simulink model "raibert_controller_walking"  (R2018b)
settings: Solver=FixedStepDiscrete  StartTime=0.0  StopTime=inf  FixedStep=sample_time  RelTol=1e-3
InitFcn:
  | warning off all
undefined symbols (not defined in the file or in its folder): ctrl, DiscIntNeverNeededParam, Discrete, initial_dx_estimate, initial_dy_estimate, initial_dz_estimate, initial_z_estimate, sample_time, Time
libraries: simulink x28, ctrlSharedLib x7
(part 3 of 4)

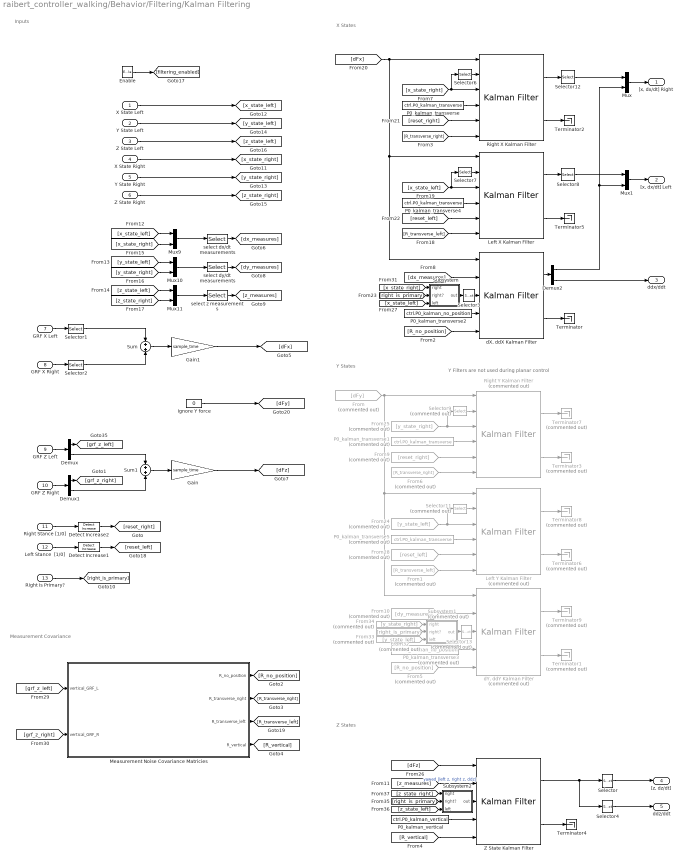
== system raibert_controller_walking/Behavior/Filtering/Kalman Filtering ==
  note: Y Filters are not used during planar control
  note: Inputs
  note: X States
  note: Y States
  note: Z States
  note: Measurement Covariance
  X State Left : Inport  SampleTime=sample_time
  Y State Left : Inport  Port=2  SampleTime=sample_time
  Z State Left : Inport  Port=3  SampleTime=sample_time
  X State Right : Inport  Port=4  SampleTime=sample_time
  Y State Right : Inport  Port=5  SampleTime=sample_time
  Z State Right : Inport  Port=6  SampleTime=sample_time
  GRF X Left : Inport  Port=7  SampleTime=sample_time
  GRF X Right : Inport  Port=8  SampleTime=sample_time
  GRF Z Left : Inport  Port=9  SampleTime=sample_time
  GRF Z Right : Inport  Port=10  SampleTime=sample_time
  Right Stance [1/0] : Inport  Port=11  PortDimensions=1  SampleTime=sample_time
  Left Stance  [1/0] : Inport  Port=12  PortDimensions=1  SampleTime=sample_time
  Right Is Primary? : Inport  Port=13  SampleTime=sample_time
  Enable : EnablePort  StatesWhenEnabling=reset  ShowOutputPort=on
  Demux : Demux  Outputs=2
  Demux1 : Demux  Outputs=2
  Demux2 : Demux  Outputs=2
  Detect Increase1 : simulink/Logic and Bit Operations/Detect Increase  vinit=0.0  OutDataTypeStr=boolean
  Detect Increase2 : simulink/Logic and Bit Operations/Detect Increase  vinit=0.0  OutDataTypeStr=boolean
  From : From  Commented=on  GotoTag=dFy
  From1 : From  Commented=on  GotoTag=R_transverse_left
  From10 : From  Commented=on  GotoTag=dy_measures
  From24 : From  Commented=on  GotoTag=y_state_left
  From25 : From  Commented=on  GotoTag=y_state_right
  From28 : From  Commented=on  GotoTag=reset_left
  From32 : From  Commented=on  GotoTag=right_is_primary
  From33 : From  Commented=on  GotoTag=y_state_left
  From34 : From  Commented=on  GotoTag=y_state_right
  From5 : From  Commented=on  GotoTag=R_no_position
  From6 : From  Commented=on  GotoTag=R_transverse_right
  From9 : From  Commented=on  GotoTag=reset_right
  Gain : Gain  Gain=sample_time
  Gain1 : Gain  Gain=sample_time
  Ignore Y force : Constant  Value=0
  Left X Kalman Filter : ctrlSharedLib/Kalman Filter  TimeDomain=Discrete-Time  UseCurrentEstimator=on  ModelSource=Individual A, B, C, D matrices  ModelSourceVariable=A_kf  A=ctrl.A_kalman_3rd_order  B=ctrl.B_kalman_3rd_order  C=ctrl.C_kalman_transverse  D=0  NumberOfStates=2  NumberOfInputs=1  NumberOfOutputs=2  InitialEstimateSource=Input port  X0=initial_dx_estimate  P0=P0_kalman_transverse  UseK=off  UseGH=on  NumberOfProcessNoiseInputs=1  G=ctrl.G_kalman_transverse  TimeInvariantG=on  H=0  TimeInvariantH=on  Q=ctrl.Q_kalman_GRFx_difference*sample_time  TimeInvariantQ=on  R=1  TimeInvariantR=off  N=0  TimeInvariantN=on  AddInputPort=on  AddEnablePort=off  ExternalReset=Rising  OutputEstimatedY=off  OutputP=on  Ts=sample_time
      settings: SourceProductBaseCode=CT
  Left Y Kalman Filter : ctrlSharedLib/Kalman Filter  Commented=on  TimeDomain=Discrete-Time  UseCurrentEstimator=on  ModelSource=Individual A, B, C, D matrices  ModelSourceVariable=A_kf  A=ctrl.A_kalman_3rd_order  B=ctrl.B_kalman_3rd_order  C=ctrl.C_kalman_transverse  D=0  NumberOfStates=2  NumberOfInputs=1  NumberOfOutputs=2  InitialEstimateSource=Input port  X0=initial_dy_estimate  P0=P0_kalman_transverse  UseK=off  UseGH=on  NumberOfProcessNoiseInputs=1  G=ctrl.G_kalman_transverse  TimeInvariantG=on  H=0  TimeInvariantH=on  Q=ctrl.Q_kalman_GRFy_difference*sample_time  TimeInvariantQ=on  R=1  TimeInvariantR=off  N=0  TimeInvariantN=on  AddInputPort=on  AddEnablePort=off  ExternalReset=Rising  OutputEstimatedY=off  OutputP=on  Ts=sample_time
      settings: SourceProductBaseCode=CT
  Measurement Noise Covariance Matricies : MATLAB Function  TreatAsAtomicUnit=on
  Mux{,1,9..11} (5 alike) : Mux  Inputs=2
  P0_kalman_transverse : Constant  Value=ctrl.P0_kalman_transverse
  P0_kalman_transverse1 : Constant  Commented=on  Value=ctrl.P0_kalman_transverse
  P0_kalman_transverse2 : Constant  Value=ctrl.P0_kalman_no_position
  P0_kalman_transverse3 : Constant  Commented=on  Value=ctrl.P0_kalman_no_position
  P0_kalman_transverse4 : Constant  Value=ctrl.P0_kalman_transverse
  P0_kalman_transverse5 : Constant  Commented=on  Value=ctrl.P0_kalman_transverse
  P0_kalman_vertical : Constant  Value=ctrl.P0_kalman_vertical
  Right X Kalman Filter : ctrlSharedLib/Kalman Filter  TimeDomain=Discrete-Time  UseCurrentEstimator=on  ModelSource=Individual A, B, C, D matrices  ModelSourceVariable=A_kf  A=ctrl.A_kalman_3rd_order  B=ctrl.B_kalman_3rd_order  C=ctrl.C_kalman_transverse  D=0  NumberOfStates=2  NumberOfInputs=1  NumberOfOutputs=2  InitialEstimateSource=Input port  X0=initial_dx_estimate  P0=P0_kalman_transverse  UseK=off  UseGH=on  NumberOfProcessNoiseInputs=1  G=ctrl.G_kalman_transverse  TimeInvariantG=on  H=0  TimeInvariantH=on  Q=ctrl.Q_kalman_GRFx_difference*sample_time  TimeInvariantQ=on  R=1  TimeInvariantR=off  N=0  TimeInvariantN=on  AddInputPort=on  AddEnablePort=off  ExternalReset=Rising  OutputEstimatedY=off  OutputP=on  Ts=sample_time
      settings: SourceProductBaseCode=CT
  Right Y Kalman Filter : ctrlSharedLib/Kalman Filter  Commented=on  TimeDomain=Discrete-Time  UseCurrentEstimator=on  ModelSource=Individual A, B, C, D matrices  ModelSourceVariable=A_kf  A=ctrl.A_kalman_3rd_order  B=ctrl.B_kalman_3rd_order  C=ctrl.C_kalman_transverse  D=0  NumberOfStates=2  NumberOfInputs=1  NumberOfOutputs=2  InitialEstimateSource=Input port  X0=initial_dy_estimate  P0=P0_kalman_transverse  UseK=off  UseGH=on  NumberOfProcessNoiseInputs=1  G=ctrl.G_kalman_transverse  TimeInvariantG=on  H=0  TimeInvariantH=on  Q=ctrl.Q_kalman_GRFy_difference*sample_time  TimeInvariantQ=on  R=1  TimeInvariantR=off  N=0  TimeInvariantN=on  AddInputPort=on  AddEnablePort=off  ExternalReset=Rising  OutputEstimatedY=off  OutputP=on  Ts=sample_time
      settings: SourceProductBaseCode=CT
  Selector : Selector  InputPortWidth=3  IndexOptions=Index vector (dialog)  Indices=[1 2]  OutputSizes=1
  Selector1 : Selector  InputPortWidth=2  IndexOptions=Index vector (dialog)  Indices=[2]  OutputSizes=1
  Selector11 : Selector  Commented=on  InputPortWidth=3  IndexOptions=Index vector (dialog)  Indices=[1 3]  OutputSizes=1
  Selector12 : Selector  InputPortWidth=3  IndexOptions=Index vector (dialog)  Indices=[1]  OutputSizes=1
  Selector13 : Selector  Commented=on  InputPortWidth=3  IndexOptions=Index vector (dialog)  Indices=[2 3]  OutputSizes=1
  Selector2 : Selector  InputPortWidth=2  IndexOptions=Index vector (dialog)  Indices=[2]  OutputSizes=1
  Selector3 : Selector  InputPortWidth=3  IndexOptions=Index vector (dialog)  Indices=[2 3]  OutputSizes=1
  Selector4 : Selector  InputPortWidth=3  IndexOptions=Index vector (dialog)  Indices=[3]  OutputSizes=1
  Selector6 : Selector  InputPortWidth=3  IndexOptions=Index vector (dialog)  Indices=[1 3]  OutputSizes=1
  Selector7 : Selector  InputPortWidth=3  IndexOptions=Index vector (dialog)  Indices=[1 3]  OutputSizes=1
  Selector8 : Selector  InputPortWidth=3  IndexOptions=Index vector (dialog)  Indices=[1]  OutputSizes=1
  Selector9 : Selector  Commented=on  InputPortWidth=3  IndexOptions=Index vector (dialog)  Indices=[1 3]  OutputSizes=1
  Subsystem : Subsystem
  Subsystem1 : Subsystem  Commented=on
  Subsystem2 : Subsystem
  Sum : Sum  Inputs=+|+
  Sum1 : Sum  Inputs=+|+
  Terminator{,2,4..5} (4 alike) : Terminator
  Terminator{1,3,6..9} (6 alike) : Terminator  Commented=on
  Z State Kalman Filter : ctrlSharedLib/Kalman Filter  TimeDomain=Discrete-Time  UseCurrentEstimator=on  ModelSource=Individual A, B, C, D matrices  ModelSourceVariable=A_kf  A=ctrl.A_kalman_3rd_order  B=ctrl.B_kalman_3rd_order  C=ctrl.C_kalman_vertical  D=0  NumberOfStates=2  NumberOfInputs=1  NumberOfOutputs=2  InitialEstimateSource=Input port  X0=[initial_z_estimate; initial_dz_estimate]  P0=P0_kalman_vertical  UseK=off  UseGH=on  NumberOfProcessNoiseInputs=1  G=ctrl.G_kalman_vertical  TimeInvariantG=on  H=0  TimeInvariantH=on  Q=ctrl.Q_kalman_GRFz_difference*sample_time  TimeInvariantQ=on  R=1  TimeInvariantR=off  N=0  TimeInvariantN=on  AddInputPort=on  AddEnablePort=off  OutputEstimatedY=off  OutputP=on  Ts=sample_time
      settings: SourceProductBaseCode=CT
  "dX, ddX Kalman Filter" : ctrlSharedLib/Kalman Filter  TimeDomain=Discrete-Time  UseCurrentEstimator=on  ModelSource=Individual A, B, C, D matrices  ModelSourceVariable=A_kf  A=ctrl.A_kalman_2nd_order  B=ctrl.B_kalman_2nd_order  C=ctrl.C_kalman_no_position  D=0  NumberOfStates=2  NumberOfInputs=1  NumberOfOutputs=2  InitialEstimateSource=Input port  X0=initial_dx_estimate  P0=P0_kalman_transverse  UseK=off  UseGH=on  NumberOfProcessNoiseInputs=1  G=ctrl.G_kalman_no_position  TimeInvariantG=on  H=0  TimeInvariantH=on  Q=ctrl.Q_kalman_GRFx_difference*sample_time  TimeInvariantQ=on  R=1  TimeInvariantR=off  N=0  TimeInvariantN=on  AddInputPort=on  AddEnablePort=off  OutputEstimatedY=off  OutputP=on  Ts=sample_time
      settings: SourceProductBaseCode=CT
  "dY, ddY Kalman Filter" : ctrlSharedLib/Kalman Filter  Commented=on  TimeDomain=Discrete-Time  UseCurrentEstimator=on  ModelSource=Individual A, B, C, D matrices  ModelSourceVariable=A_kf  A=ctrl.A_kalman_2nd_order  B=ctrl.B_kalman_2nd_order  C=ctrl.C_kalman_no_position  D=0  NumberOfStates=2  NumberOfInputs=1  NumberOfOutputs=2  InitialEstimateSource=Input port  X0=initial_dx_estimate  P0=P0_kalman_transverse  UseK=off  UseGH=on  NumberOfProcessNoiseInputs=1  G=ctrl.G_kalman_no_position  TimeInvariantG=on  H=0  TimeInvariantH=on  Q=ctrl.Q_kalman_GRFx_difference*sample_time  TimeInvariantQ=on  R=1  TimeInvariantR=off  N=0  TimeInvariantN=on  AddInputPort=on  AddEnablePort=off  OutputEstimatedY=off  OutputP=on  Ts=sample_time
      settings: SourceProductBaseCode=CT
  select dx/dt measurements : Selector  InputPortWidth=6  IndexOptions=Index vector (dialog)  Indices=[2 5 6]  OutputSizes=1
  select dy/dt measurements : Selector  InputPortWidth=6  IndexOptions=Index vector (dialog)  Indices=[2 5 6]  OutputSizes=1
  select z measurements : Selector  InputPortWidth=6  IndexOptions=Index vector (dialog)  Indices=[1 4 6]  OutputSizes=1
  "[x, dx/dt] Right" : Outport
  "[x, dx/dt] Left" : Outport  Port=2
  ddx/ddt : Outport  Port=3
  "[z, dz/dt]" : Outport  Port=4
  ddz/ddt : Outport  Port=5
  wires:
  [R_no_position] -> "dX, ddX Kalman Filter"/5
  P0_kalman_transverse2/1 -> "dX, ddX Kalman Filter"/4
  Subsystem/1(out) -> Selector3/1
  [dx_measures] -> "dX, ddX Kalman Filter"/2
  Z State Kalman Filter/1 -> Selector4/1, Selector/1
  [z_measures] -> Z State Kalman Filter/2  "yawed [left z, right z, ddz]"
  [R_vertical] -> Z State Kalman Filter/5
  [grf_z_right] -> Measurement Noise Covariance Matricies/2(vertical_GRF_R)
  [grf_z_left] -> Measurement Noise Covariance Matricies/1(vertical_GRF_L)
  P0_kalman_transverse1/1 -> Right Y Kalman Filter/4
  [dFz] -> Z State Kalman Filter/1
  P0_kalman_transverse/1 -> Right X Kalman Filter/4
  [dFx] -> Right X Kalman Filter/1, Left X Kalman Filter/1, "dX, ddX Kalman Filter"/1
  Right X Kalman Filter/1 -> Selector12/1
  "dX, ddX Kalman Filter"/2 -> Terminator/1
  [R_transverse_right] -> Right X Kalman Filter/6
  P0_kalman_vertical/1 -> Z State Kalman Filter/4
  "dY, ddY Kalman Filter"/2 -> Terminator1/1
  Subsystem1/1(out) -> Selector13/1
  P0_kalman_transverse3/1 -> "dY, ddY Kalman Filter"/4
  From10/1 -> "dY, ddY Kalman Filter"/2
  Measurement Noise Covariance Matricies/1(R_no_position) -> [R_no_position]
  Measurement Noise Covariance Matricies/2(R_transverse_right) -> [R_transverse_right]
  Measurement Noise Covariance Matricies/4(R_vertical) -> [R_vertical]
  From5/1 -> "dY, ddY Kalman Filter"/5
  From6/1 -> Right Y Kalman Filter/6
  Right Is Primary?/1 -> [right_is_primary]
  Y State Right/1 -> [y_state_right]
  [x_state_left] -> Mux9/1
  [x_state_right] -> Mux9/2
  [y_state_left] -> Mux10/1
  [y_state_right] -> Mux10/2
  [z_state_left] -> Mux11/1
  [z_state_right] -> Mux11/2
  Mux9/1 -> select dx/dt measurements/1
  Mux10/1 -> select dy/dt measurements/1
  Mux11/1 -> select z measurements/1
  select dx/dt measurements/1 -> [dx_measures]
  select dy/dt measurements/1 -> [dy_measures]
  select z measurements/1 -> [z_measures]
  Right X Kalman Filter/2 -> Terminator2/1
  Right Y Kalman Filter/2 -> Terminator3/1
  Z State Kalman Filter/2 -> Terminator4/1
  Enable/1 -> [filtering_enabled]
  [x_state_right] -> Selector6/1, Right X Kalman Filter/3
  Selector6/1 -> Right X Kalman Filter/2
  Selector7/1 -> Left X Kalman Filter/2
  [x_state_left] -> Left X Kalman Filter/3, Selector7/1
  [R_transverse_left] -> Left X Kalman Filter/6
  P0_kalman_transverse4/1 -> Left X Kalman Filter/4
  Left X Kalman Filter/1 -> Selector8/1
  Left X Kalman Filter/2 -> Terminator5/1
  [reset_right] -> Right X Kalman Filter/5
  [reset_left] -> Left X Kalman Filter/5
  From9/1 -> Right Y Kalman Filter/5
  From25/1 -> Selector9/1, Right Y Kalman Filter/3
  Selector9/1 -> Right Y Kalman Filter/2
  Selector11/1 -> Left Y Kalman Filter/2
  From24/1 -> Left Y Kalman Filter/3, Selector11/1
  From28/1 -> Left Y Kalman Filter/5
  Left Y Kalman Filter/2 -> Terminator6/1
  From1/1 -> Left Y Kalman Filter/6
  From/1 -> Right Y Kalman Filter/1, Left Y Kalman Filter/1, "dY, ddY Kalman Filter"/1
  P0_kalman_transverse5/1 -> Left Y Kalman Filter/4
  Right Stance [1/0]/1 -> Detect Increase2/1
  Left Stance  [1/0]/1 -> Detect Increase1/1
  Detect Increase1/1 -> [reset_left]
  Detect Increase2/1 -> [reset_right]
  GRF X Left/1 -> Selector1/1
  GRF X Right/1 -> Selector2/1
  Sum/1 -> Gain1/1
  Measurement Noise Covariance Matricies/3(R_transverse_left) -> [R_transverse_left]
  GRF Z Left/1 -> Demux/1
  GRF Z Right/1 -> Demux1/1
  Sum1/1 -> Gain/1
  Demux/1 -> [grf_z_left]
  Demux1/1 -> [grf_z_right]
  Selector1/1 -> Sum/1
  Selector2/1 -> Sum/2
  Demux/2 -> Sum1/1
  Demux1/2 -> Sum1/2
  Gain/1 -> [dFz]
  Gain1/1 -> [dFx]
  Ignore Y force/1 -> [dFy]
  Mux/1 -> "[x, dx/dt] Right"/1
  Selector12/1 -> Mux/1
  Mux1/1 -> "[x, dx/dt] Left"/1
  Selector8/1 -> Mux1/1
  Right Y Kalman Filter/1 -> Terminator7/1
  Left Y Kalman Filter/1 -> Terminator8/1
  "dY, ddY Kalman Filter"/1 -> Terminator9/1
  [x_state_right] -> Subsystem/1(right)
  [right_is_primary] -> Subsystem/2(right?)
  [x_state_left] -> Subsystem/3(left)
  From32/1 -> Subsystem1/2(right?)
  From34/1 -> Subsystem1/1(right)
  From33/1 -> Subsystem1/3(left)
  Selector13/1 -> "dY, ddY Kalman Filter"/3
  Selector3/1 -> "dX, ddX Kalman Filter"/3
  [right_is_primary] -> Subsystem2/2(right?)
  [z_state_right] -> Subsystem2/1(right)
  [z_state_left] -> Subsystem2/3(left)
  Subsystem2/1(out) -> Z State Kalman Filter/3
  Selector/1 -> "[z, dz/dt]"/1
  Demux2/1 -> Mux1/2, Mux/2
  Demux2/2 -> ddx/ddt/1
  Selector4/1 -> ddz/ddt/1
  "dX, ddX Kalman Filter"/1 -> Demux2/1
  Z State Left/1 -> [z_state_left]
  Y State Left/1 -> [y_state_left]
  X State Left/1 -> [x_state_left]
  Z State Right/1 -> [z_state_right]
  X State Right/1 -> [x_state_right]

== system raibert_controller_walking/Behavior/Filtering/Subsystem2 ==
  right : Inport
  right? : Inport  Port=2
  left : Inport  Port=3
  Switch : Switch  Criteria=u2 ~= 0
  out : Outport
  wires:
  right/1 -> Switch/1
  right?/1 -> Switch/2
  left/1 -> Switch/3
  Switch/1 -> out/1

== system raibert_controller_walking/Behavior/Raibert Controller/Hold Value ==
  In : Inport
  Enable : EnablePort
  Out : Outport  InitialOutput=0
  wires:
  In/1 -> Out/1

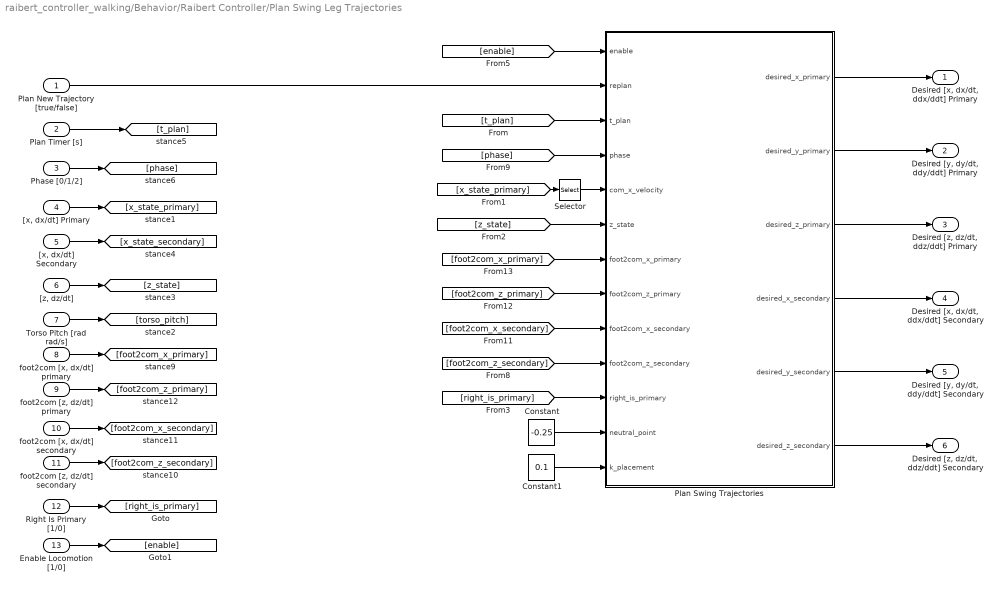
== system raibert_controller_walking/Behavior/Raibert Controller/Plan Swing Leg Trajectories ==
  Plan New Trajectory [true/false] : Inport
  Plan Timer [s] : Inport  Port=2
  Phase [0/1/2] : Inport  Port=3
  "[x, dx/dt] Primary" : Inport  Port=4
  "[x, dx/dt] Secondary" : Inport  Port=5
  "[z, dz/dt]" : Inport  Port=6
  Torso Pitch [rad rad/s] : Inport  Port=7
  "foot2com [x, dx/dt] primary" : Inport  Port=8
  "foot2com [z, dz/dt] primary" : Inport  Port=9
  "foot2com [x, dx/dt] secondary" : Inport  Port=10
  "foot2com [z, dz/dt] secondary" : Inport  Port=11
  Right Is Primary [1/0] : Inport  Port=12
  Enable Locomotion [1/0] : Inport  Port=13
  Constant : Constant  Value=-0.25
  Constant1 : Constant  Value=0.1
  Plan Swing Trajectories : MATLAB Function  TreatAsAtomicUnit=on
  Selector : Selector  InputPortWidth=2  IndexOptions=Index vector (dialog)  Indices=[2]  OutputSizes=1
  "Desired [x, dx/dt, ddx/ddt] Primary" : Outport
  "Desired [y, dy/dt, ddy/ddt] Primary" : Outport  Port=2
  "Desired [z, dz/dt, ddz/ddt] Primary" : Outport  Port=3
  "Desired [x, dx/dt, ddx/ddt] Secondary" : Outport  Port=4
  "Desired [y, dy/dt, ddy/ddt] Secondary" : Outport  Port=5
  "Desired [z, dz/dt, ddz/ddt] Secondary" : Outport  Port=6
  wires:
  Plan Timer [s]/1 -> [t_plan]
  Phase [0/1/2]/1 -> [phase]
  "[x, dx/dt] Secondary"/1 -> [x_state_secondary]
  Plan New Trajectory [true/false]/1 -> Plan Swing Trajectories/2(replan)
  Torso Pitch [rad rad/s]/1 -> [torso_pitch]
  "[x, dx/dt] Primary"/1 -> [x_state_primary]
  "[z, dz/dt]"/1 -> [z_state]
  Plan Swing Trajectories/1(desired_x_primary) -> "Desired [x, dx/dt, ddx/ddt] Primary"/1
  Plan Swing Trajectories/2(desired_y_primary) -> "Desired [y, dy/dt, ddy/ddt] Primary"/1
  Plan Swing Trajectories/3(desired_z_primary) -> "Desired [z, dz/dt, ddz/ddt] Primary"/1
  Plan Swing Trajectories/4(desired_x_secondary) -> "Desired [x, dx/dt, ddx/ddt] Secondary"/1
  Plan Swing Trajectories/5(desired_y_secondary) -> "Desired [y, dy/dt, ddy/ddt] Secondary"/1
  Plan Swing Trajectories/6(desired_z_secondary) -> "Desired [z, dz/dt, ddz/ddt] Secondary"/1
  Right Is Primary [1/0]/1 -> [right_is_primary]
  Enable Locomotion [1/0]/1 -> [enable]
  "foot2com [x, dx/dt] secondary"/1 -> [foot2com_x_secondary]
  "foot2com [x, dx/dt] primary"/1 -> [foot2com_x_primary]
  "foot2com [z, dz/dt] secondary"/1 -> [foot2com_z_secondary]
  "foot2com [z, dz/dt] primary"/1 -> [foot2com_z_primary]
  [enable] -> Plan Swing Trajectories/1(enable)
  [t_plan] -> Plan Swing Trajectories/3(t_plan)
  [phase] -> Plan Swing Trajectories/4(phase)
  [z_state] -> Plan Swing Trajectories/6(z_state)
  [foot2com_x_primary] -> Plan Swing Trajectories/7(foot2com_x_primary)
  [foot2com_z_primary] -> Plan Swing Trajectories/8(foot2com_z_primary)
  [foot2com_x_secondary] -> Plan Swing Trajectories/9(foot2com_x_secondary)
  [foot2com_z_secondary] -> Plan Swing Trajectories/10(foot2com_z_secondary)
  [right_is_primary] -> Plan Swing Trajectories/11(right_is_primary)
  [x_state_primary] -> Selector/1
  Selector/1 -> Plan Swing Trajectories/5(com_x_velocity)
  Constant/1 -> Plan Swing Trajectories/12(neutral_point)
  Constant1/1 -> Plan Swing Trajectories/13(k_placement)

== system raibert_controller_walking/Behavior/Raibert Controller/Stance Control ==
  "[z, dz/dt]" : Inport
  "Torso Pitch [rad, rad/s]" : Inport  Port=2
  "[x, dx/dt] Primary" : Inport  Port=3
  In Double? : Inport  Port=4
  Enable Locomotion : Inport  Port=5
  BoundFx : Fcn  Expr=u(1)
  Constant1 : Constant  Value=[0; 0]
  Constant2 : Constant  Value=true
  Constant3 : Constant  Value=ctrl.torso_pitch_desired
  Data Type Conversion : DataTypeConversion  OutDataTypeStr=double
  Discrete-Time Integrator : DiscreteIntegrator  Commented=on  gainval=1  SampleTime=-1  ICPrevOutput=DiscIntNeverNeededParam  ICPrevScaledInput=DiscIntNeverNeededParam
  Divide : Product  Inputs=*/*
  Fx : Fcn  Expr=ctrl.kp_theta*(u(1) - ctrl.torso_pitch_desired) + ctrl.ki_theta*u(3) +ctrl.kd_theta*(u(2)) + ctrl.kp_x*(-u(4)) + ctrl.kd_x*(ctrl.com_x_vel_desired - u(5))
  Fz : Fcn  Expr=ctrl.weight_factor*ctrl.m_total*ctrl.g + ctrl.kp_z*(ctrl.z_com_desired - u(1)) - ctrl.kd_z*(u(2))
  Gain : Gain  Gain=0
  Logical Operator : Logic  AllPortsSameDT=off  OutDataTypeStr=boolean
  Mux : Mux  Inputs=2
  Mux1 : Mux  Inputs=2
  Mux3 : Mux  Inputs=3
  NOT : Logic  Operator=NOT  IconShape=distinctive  AllPortsSameDT=off  OutDataTypeStr=boolean
  Product : Product
  Product1 : Product
  Selector : Selector  InputPortWidth=2  IndexOptions=Index vector (dialog)  Indices=[1]  OutputSizes=1
  Selector1 : Selector  InputPortWidth=2  IndexOptions=Index vector (dialog)  Indices=[1]  OutputSizes=1
  Selector2 : Selector  InputPortWidth=2  IndexOptions=Index vector (dialog)  Indices=[1]  OutputSizes=1
  Sum : Sum  Inputs=++|
  Sum1 : Sum  Inputs=|+-
  Desired [Fx Fz] Primary : Outport
  Desired [Fx Fz] Secondary : Outport  Port=2
  wires:
  Constant1/1 -> Desired [Fx Fz] Secondary/1
  "[z, dz/dt]"/1 -> Selector1/1, Fz/1
  Mux/1 -> Desired [Fx Fz] Primary/1
  In Double?/1 -> NOT/1
  Logical Operator/1 -> Data Type Conversion/1
  Data Type Conversion/1 -> Product/1, Product1/2
  Product/1 -> Mux/2
  Product1/1 -> Mux/1
  Fx/1 -> Sum/1
  Fz/1 -> Divide/3, Mux1/2, Product/2
  Selector/1 -> Divide/1
  Selector1/1 -> Divide/2
  Divide/1 -> Sum/2
  Sum/1 -> Mux1/1
  Mux1/1 -> BoundFx/1
  BoundFx/1 -> Product1/1
  NOT/1 -> Logical Operator/2
  Sum1/1 -> Gain/1
  Gain/1 -> Mux3/2
  Mux3/1 -> Fx/1
  "Torso Pitch [rad, rad/s]"/1 -> Selector2/1, Mux3/1
  "[x, dx/dt] Primary"/1 -> Mux3/3, Selector/1
  Constant3/1 -> Sum1/2
  Selector2/1 -> Sum1/1
  Constant2/1 -> Logical Operator/1

== system raibert_controller_walking/Behavior/Swing Leg Control Primary/Back//Front PD (torque) ==
  Desired Position [rad] [back front] : Inport
  Desired Velocity [rad/s] [back front] : Inport  Port=2
  Desired Acceleration [rad/s^2] [back front] : Inport  Port=3
  Measured Position [rad] [back front] : Inport  Port=4
  Measured Velocity [rad/s] [back front] : Inport  Port=5
  Back / Front Position Tracking : Scope  NumInputPorts=2
  Back / Front Velocity Tracking : Scope  NumInputPorts=2
  Feedback / Feedforward : Scope  NumInputPorts=2
  Kp_SEA_Trajectory : Constant  Value=ctrl.kp_torque_swing
  Kp_SEA_Trajectory1 : Constant  Value=ctrl.kd_torque_swing
  Kp_SEA_Trajectory2 : Constant  Value=ctrl.i_motor
  Mux{1..2,12..13} (4 alike) : Mux  Inputs=2
  Product1 : Product
  Product2 : Product
  Product3 : Product
  Selector{,1..3} (4 alike) : Selector  InputPortWidth=2  IndexOptions=Index vector (dialog)  Indices=[1]  OutputSizes=1
  Selector{4..5,7..8} (4 alike) : Selector  InputPortWidth=2  IndexOptions=Index vector (dialog)  Indices=[2]  OutputSizes=1
  Sum1 : Sum  Inputs=|+-
  Sum2 : Sum  Inputs=|++
  Sum7 : Sum  Inputs=|+-
  Sum9 : Sum  Inputs=++|
  Commanded Torque [Nm] [back front] : Outport
  wires:
  Product3/1 -> Sum2/2, Feedback / Feedforward/2
  Kp_SEA_Trajectory2/1 -> Product3/1
  Desired Acceleration [rad/s^2] [back front]/1 -> Product3/2
  Sum2/1 -> Commanded Torque [Nm] [back front]/1
  Sum9/1 -> Sum2/1, Feedback / Feedforward/1
  Kp_SEA_Trajectory1/1 -> Product2/2
  Sum1/1 -> Product2/1
  Kp_SEA_Trajectory/1 -> Product1/2
  Measured Position [rad] [back front]/1 -> Selector4/1, Selector/1, Sum7/2
  Sum7/1 -> Product1/1
  Product1/1 -> Sum9/1
  Mux13/1 -> Back / Front Position Tracking/1
  Desired Position [rad] [back front]/1 -> Selector5/1, Selector1/1, Sum7/1
  Mux2/1 -> Back / Front Position Tracking/2
  Selector/1 -> Mux13/1
  Selector1/1 -> Mux13/2
  Selector5/1 -> Mux2/2
  Selector4/1 -> Mux2/1
  Desired Velocity [rad/s] [back front]/1 -> Selector8/1, Selector3/1, Sum1/1
  Product2/1 -> Sum9/2
  Measured Velocity [rad/s] [back front]/1 -> Sum1/2, Selector2/1, Selector7/1
  Mux1/1 -> Back / Front Velocity Tracking/1
  Selector2/1 -> Mux1/1
  Selector7/1 -> Mux12/1
  Mux12/1 -> Back / Front Velocity Tracking/2
  Selector8/1 -> Mux12/2
  Selector3/1 -> Mux1/2

== system raibert_controller_walking/Behavior/Swing Leg Control Primary/Back//Front PD (velocity) ==
  Desired Position [rad] [back front] : Inport
  Desired Velocity [rad/s] [back front] : Inport  Port=2
  Desired Acceleration [rad/s^2] [back front] : Inport  Port=3
  Measured Position [rad] [back front] : Inport  Port=4
  Measured Velocity [rad/s] [back front] : Inport  Port=5
  Back / Front PositionTracking : Scope  NumInputPorts=2
  Back / Front Velocity Tracking : Scope  NumInputPorts=2
  Feedback / Feedforward : Scope  NumInputPorts=2
  Feedforward Gain : Gain
  Kp_SEA_Trajectory : Constant  Value=ctrl.kp_velocity_swing
  Mux{1..2,12..13} (4 alike) : Mux  Inputs=2
  Product1 : Product
  Selector{,1..3} (4 alike) : Selector  InputPortWidth=2  IndexOptions=Index vector (dialog)  Indices=[1]  OutputSizes=1
  Selector{4..5,7..8} (4 alike) : Selector  InputPortWidth=2  IndexOptions=Index vector (dialog)  Indices=[2]  OutputSizes=1
  Sum7 : Sum  Inputs=|+-
  Sum9 : Sum
  Terminator : Terminator
  Commanded Velocity [rad/s] [back front] : Outport
  wires:
  Selector3/1 -> Mux1/2
  Selector8/1 -> Mux12/2
  Mux12/1 -> Back / Front Velocity Tracking/2
  Selector7/1 -> Mux12/1
  Selector2/1 -> Mux1/1
  Mux1/1 -> Back / Front Velocity Tracking/1
  Measured Velocity [rad/s] [back front]/1 -> Selector2/1, Selector7/1
  Desired Acceleration [rad/s^2] [back front]/1 -> Terminator/1
  Feedforward Gain/1 -> Sum9/2, Feedback / Feedforward/2
  Desired Velocity [rad/s] [back front]/1 -> Selector3/1, Selector8/1, Feedforward Gain/1
  Selector4/1 -> Mux2/1
  Selector5/1 -> Mux2/2
  Selector1/1 -> Mux13/2
  Selector/1 -> Mux13/1
  Mux2/1 -> Back / Front PositionTracking/2
  Desired Position [rad] [back front]/1 -> Sum7/1, Selector1/1, Selector5/1
  Mux13/1 -> Back / Front PositionTracking/1
  Product1/1 -> Sum9/1, Feedback / Feedforward/1
  Sum7/1 -> Product1/1
  Measured Position [rad] [back front]/1 -> Sum7/2, Selector/1, Selector4/1
  Sum9/1 -> Commanded Velocity [rad/s] [back front]/1
  Kp_SEA_Trajectory/1 -> Product1/2

== system raibert_controller_walking/Behavior/Swing Leg Control Primary/Lateral PD (torque) ==
  note: (Approximation)
      | This is the lateral torque generated due to the relative
      | acceleration of the motor around the pelvis. Only
      | approximate vertical components are used in the
      | calculation. The lateral components are small.
  Desired Position [rad] : Inport
  Desired Velocity [rad/s] : Inport  Port=2
  Desired Acceleration [rad/s^2] : Inport  Port=3
  Measured Position [rad] : Inport  Port=4
  Measured Velocity [rad/s] : Inport  Port=5
  CoM Z Acceleration [m/s^2] : Inport  Port=6
  Feedback / Feedforward : Scope  NumInputPorts=2
  Kp_SEA_Trajectory : Constant  Value=ctrl.kp_lateral_swing
  Kp_SEA_Trajectory1 : Constant  Value=ctrl.kd_lateral_swing
  Kp_SEA_Trajectory2 : Constant  Value=ctrl.i_lateral_about_pelvis
  Kp_SEA_Trajectory3 : Constant  Value=ctrl.lateral_offset
  Kp_SEA_Trajectory4 : Constant  Value=(ctrl.m_leg_motor + ctrl.m_leg)
  Kp_SEA_Trajectory5 : Constant  Value=-ctrl.g
  Mux13 : Mux  Inputs=2
  Mux2 : Mux  Inputs=2
  Position / Velocity Tracking : Scope  NumInputPorts=2
  Product1 : Product
  Product2 : Product
  Product3 : Product
  Product4 : Product  Inputs=3
  Sum1 : Sum  Inputs=|+-
  Sum2 : Sum  Inputs=|++
  Sum3 : Sum  Inputs=|++
  Sum4 : Sum  Inputs=|+-
  Sum7 : Sum  Inputs=|+-
  Sum9 : Sum  Inputs=++|
  Commanded Torque [Nm] : Outport
  wires:
  Sum4/1 -> Product4/1
  CoM Z Acceleration [m/s^2]/1 -> Sum4/2
  Kp_SEA_Trajectory5/1 -> Sum4/1
  Kp_SEA_Trajectory3/1 -> Product4/2
  Kp_SEA_Trajectory4/1 -> Product4/3
  Product4/1 -> Sum3/2
  Product3/1 -> Sum3/1
  Measured Velocity [rad/s]/1 -> Sum1/2, Mux2/1
  Product2/1 -> Sum9/2
  Desired Velocity [rad/s]/1 -> Sum1/1, Mux2/2
  Mux2/1 -> Position / Velocity Tracking/2
  Desired Position [rad]/1 -> Sum7/1, Mux13/2
  Mux13/1 -> Position / Velocity Tracking/1
  Product1/1 -> Sum9/1
  Sum7/1 -> Product1/1
  Measured Position [rad]/1 -> Sum7/2, Mux13/1
  Kp_SEA_Trajectory/1 -> Product1/2
  Sum1/1 -> Product2/1
  Kp_SEA_Trajectory1/1 -> Product2/2
  Sum9/1 -> Feedback / Feedforward/1, Sum2/1
  Sum2/1 -> Commanded Torque [Nm]/1
  Desired Acceleration [rad/s^2]/1 -> Product3/2
  Kp_SEA_Trajectory2/1 -> Product3/1
  Sum3/1 -> Feedback / Feedforward/2, Sum2/2

== system raibert_controller_walking/Behavior/Swing Leg Control Secondary/Back//Front PD (torque) ==
  Desired Position [rad] [back front] : Inport
  Desired Velocity [rad/s] [back front] : Inport  Port=2
  Desired Acceleration [rad/s^2] [back front] : Inport  Port=3
  Measured Position [rad] [back front] : Inport  Port=4
  Measured Velocity [rad/s] [back front] : Inport  Port=5
  Back / Front Position Tracking : Scope  NumInputPorts=2
  Back / Front Velocity Tracking : Scope  NumInputPorts=2
  Feedback / Feedforward : Scope  NumInputPorts=2
  Kp_SEA_Trajectory : Constant  Value=ctrl.kp_torque_swing
  Kp_SEA_Trajectory1 : Constant  Value=ctrl.kd_torque_swing
  Kp_SEA_Trajectory2 : Constant  Value=ctrl.i_motor
  Mux{1..2,12..13} (4 alike) : Mux  Inputs=2
  Product1 : Product
  Product2 : Product
  Product3 : Product
  Selector{,1..3} (4 alike) : Selector  InputPortWidth=2  IndexOptions=Index vector (dialog)  Indices=[1]  OutputSizes=1
  Selector{4..5,7..8} (4 alike) : Selector  InputPortWidth=2  IndexOptions=Index vector (dialog)  Indices=[2]  OutputSizes=1
  Sum1 : Sum  Inputs=|+-
  Sum2 : Sum  Inputs=|++
  Sum7 : Sum  Inputs=|+-
  Sum9 : Sum  Inputs=++|
  Commanded Torque [Nm] [back front] : Outport
  wires:
  Selector3/1 -> Mux1/2
  Selector8/1 -> Mux12/2
  Mux12/1 -> Back / Front Velocity Tracking/2
  Selector7/1 -> Mux12/1
  Selector2/1 -> Mux1/1
  Mux1/1 -> Back / Front Velocity Tracking/1
  Measured Velocity [rad/s] [back front]/1 -> Selector7/1, Selector2/1, Sum1/2
  Product2/1 -> Sum9/2
  Desired Velocity [rad/s] [back front]/1 -> Sum1/1, Selector3/1, Selector8/1
  Selector4/1 -> Mux2/1
  Selector5/1 -> Mux2/2
  Selector1/1 -> Mux13/2
  Selector/1 -> Mux13/1
  Mux2/1 -> Back / Front Position Tracking/2
  Desired Position [rad] [back front]/1 -> Sum7/1, Selector1/1, Selector5/1
  Mux13/1 -> Back / Front Position Tracking/1
  Product1/1 -> Sum9/1
  Sum7/1 -> Product1/1
  Measured Position [rad] [back front]/1 -> Sum7/2, Selector/1, Selector4/1
  Kp_SEA_Trajectory/1 -> Product1/2
  Sum1/1 -> Product2/1
  Kp_SEA_Trajectory1/1 -> Product2/2
  Sum9/1 -> Feedback / Feedforward/1, Sum2/1
  Sum2/1 -> Commanded Torque [Nm] [back front]/1
  Desired Acceleration [rad/s^2] [back front]/1 -> Product3/2
  Kp_SEA_Trajectory2/1 -> Product3/1
  Product3/1 -> Sum2/2, Feedback / Feedforward/2

== system raibert_controller_walking/Behavior/Swing Leg Control Secondary/Back//Front PD (velocity) ==
  Desired Position [rad] [back front] : Inport
  Desired Velocity [rad/s] [back front] : Inport  Port=2
  Desired Acceleration [rad/s^2] [back front] : Inport  Port=3
  Measured Position [rad] [back front] : Inport  Port=4
  Measured Velocity [rad/s] [back front] : Inport  Port=5
  Back / Front PositionTracking : Scope  NumInputPorts=2
  Back / Front Velocity Tracking : Scope  NumInputPorts=2
  Feedback / Feedforward : Scope  NumInputPorts=2
  Feedforward Gain : Gain
  Kp_SEA_Trajectory : Constant  Value=ctrl.kp_velocity_swing
  Mux{1..2,12..13} (4 alike) : Mux  Inputs=2
  Product1 : Product
  Selector{,1..3} (4 alike) : Selector  InputPortWidth=2  IndexOptions=Index vector (dialog)  Indices=[1]  OutputSizes=1
  Selector{4..5,7..8} (4 alike) : Selector  InputPortWidth=2  IndexOptions=Index vector (dialog)  Indices=[2]  OutputSizes=1
  Sum7 : Sum  Inputs=|+-
  Sum9 : Sum
  Terminator : Terminator
  Commanded Velocity [rad/s] [back front] : Outport
  wires:
  Kp_SEA_Trajectory/1 -> Product1/2
  Sum9/1 -> Commanded Velocity [rad/s] [back front]/1
  Measured Position [rad] [back front]/1 -> Selector4/1, Selector/1, Sum7/2
  Sum7/1 -> Product1/1
  Product1/1 -> Feedback / Feedforward/1, Sum9/1
  Mux13/1 -> Back / Front PositionTracking/1
  Desired Position [rad] [back front]/1 -> Selector5/1, Selector1/1, Sum7/1
  Mux2/1 -> Back / Front PositionTracking/2
  Selector/1 -> Mux13/1
  Selector1/1 -> Mux13/2
  Selector5/1 -> Mux2/2
  Selector4/1 -> Mux2/1
  Desired Velocity [rad/s] [back front]/1 -> Feedforward Gain/1, Selector8/1, Selector3/1
  Feedforward Gain/1 -> Feedback / Feedforward/2, Sum9/2
  Desired Acceleration [rad/s^2] [back front]/1 -> Terminator/1
  Measured Velocity [rad/s] [back front]/1 -> Selector7/1, Selector2/1
  Mux1/1 -> Back / Front Velocity Tracking/1
  Selector2/1 -> Mux1/1
  Selector7/1 -> Mux12/1
  Mux12/1 -> Back / Front Velocity Tracking/2
  Selector8/1 -> Mux12/2
  Selector3/1 -> Mux1/2

== system raibert_controller_walking/Behavior/Swing Leg Control Secondary/Lateral PD (torque) ==
  note: (Approximation)
      | This is the lateral torque generated due to the relative
      | acceleration of the motor around the pelvis. Only
      | approximate vertical components are used in the
      | calculation. The lateral components are small.
  Desired Position [rad] : Inport
  Desired Velocity [rad/s] : Inport  Port=2
  Desired Acceleration [rad/s^2] : Inport  Port=3
  Measured Position [rad] : Inport  Port=4
  Measured Velocity [rad/s] : Inport  Port=5
  CoM Z Acceleration [m/s^2] : Inport  Port=6
  Feedback / Feedforward : Scope  NumInputPorts=2
  Kp_SEA_Trajectory : Constant  Value=ctrl.kp_lateral_swing
  Kp_SEA_Trajectory1 : Constant  Value=ctrl.kd_lateral_swing
  Kp_SEA_Trajectory2 : Constant  Value=ctrl.i_lateral_about_pelvis
  Kp_SEA_Trajectory3 : Constant  Value=ctrl.lateral_offset
  Kp_SEA_Trajectory4 : Constant  Value=(ctrl.m_leg_motor + ctrl.m_leg)
  Kp_SEA_Trajectory5 : Constant  Value=-ctrl.g
  Mux13 : Mux  Inputs=2
  Mux2 : Mux  Inputs=2
  Position / Velocity Tracking : Scope  NumInputPorts=2
  Product1 : Product
  Product2 : Product
  Product3 : Product
  Product4 : Product  Inputs=3
  Sum1 : Sum  Inputs=|+-
  Sum2 : Sum  Inputs=|++
  Sum3 : Sum  Inputs=|++
  Sum4 : Sum  Inputs=|+-
  Sum7 : Sum  Inputs=|+-
  Sum9 : Sum  Inputs=++|
  Commanded Torque [Nm] : Outport
  wires:
  Sum3/1 -> Sum2/2, Feedback / Feedforward/2
  Kp_SEA_Trajectory2/1 -> Product3/1
  Desired Acceleration [rad/s^2]/1 -> Product3/2
  Sum2/1 -> Commanded Torque [Nm]/1
  Sum9/1 -> Sum2/1, Feedback / Feedforward/1
  Kp_SEA_Trajectory1/1 -> Product2/2
  Sum1/1 -> Product2/1
  Kp_SEA_Trajectory/1 -> Product1/2
  Measured Position [rad]/1 -> Mux13/1, Sum7/2
  Sum7/1 -> Product1/1
  Product1/1 -> Sum9/1
  Mux13/1 -> Position / Velocity Tracking/1
  Desired Position [rad]/1 -> Mux13/2, Sum7/1
  Mux2/1 -> Position / Velocity Tracking/2
  Desired Velocity [rad/s]/1 -> Mux2/2, Sum1/1
  Product2/1 -> Sum9/2
  Measured Velocity [rad/s]/1 -> Mux2/1, Sum1/2
  Product3/1 -> Sum3/1
  Product4/1 -> Sum3/2
  Kp_SEA_Trajectory4/1 -> Product4/3
  Kp_SEA_Trajectory3/1 -> Product4/2
  Kp_SEA_Trajectory5/1 -> Sum4/1
  CoM Z Acceleration [m/s^2]/1 -> Sum4/2
  Sum4/1 -> Product4/1

== system raibert_controller_walking/Behavior/Tranform Sensor Measurements to CoM Acceleration Measurement/Compute Body Frame Accelerations ==
  imu accelerations x3 : Inport
  IMU Accel Unfiltered vs Filtered : Scope  NumInputPorts=3
  IMU Two Pole Filter2 : DiscreteTransferFcn  Commented=on  Numerator=[ctrl.A_lpf_accelerometer 0 0]  Denominator=[1 ctrl.B1_lpf_accelerometer ctrl.B2_lpf_accelerometer]  SampleTime=sample_time
  Mux : Mux  Inputs=2
  Selector : Selector  InputPortWidth=6  IndexOptions=Index vector (dialog)  Indices=[1 4]  OutputSizes=1
  Selector1 : Selector  InputPortWidth=6  IndexOptions=Index vector (dialog)  Indices=[2 5]  OutputSizes=1
  Selector2 : Selector  InputPortWidth=6  IndexOptions=Index vector (dialog)  Indices=[3 6]  OutputSizes=1
  accelerations [m/s^2] x3 : Outport
  wires:
  Mux/1 -> Selector/1, Selector2/1, Selector1/1
  imu accelerations x3/1 -> Mux/2, accelerations [m/s^2] x3/1, Mux/1
  Selector/1 -> IMU Accel Unfiltered vs Filtered/1
  Selector1/1 -> IMU Accel Unfiltered vs Filtered/2
  Selector2/1 -> IMU Accel Unfiltered vs Filtered/3

== system raibert_controller_walking/Behavior/Tranform Sensor Measurements to CoM Acceleration Measurement/Estimate Angular Accelerations2 ==
  Angular Velocities [rad/s] x3 : Inport
  Enabled : Inport  Port=2
  Detect Change : simulink/Logic and Bit Operations/Detect Change  vinit=0  OutDataTypeStr=boolean
  Difference : simulink/Discrete/Difference  ICPrevInput=0.0  OutMin=[]  OutMax=[]  OutDataType=fixdt(1, 16)  OutScaling=2^-10  DoSatur=off
  Gain : Gain  Gain=1/sample_time
  IMU Two Pole Filter : DiscreteTransferFcn  Commented=on  Numerator=[ctrl.A_lpf_lateral_accel 0 0]  Denominator=[1 ctrl.B1_lpf_lateral_accel ctrl.B2_lpf_lateral_accel]  SampleTime=sample_time
  Logical Operator5 : Logic  Operator=NOT  AllPortsSameDT=off  OutDataTypeStr=boolean
  Product : Product
  Angular Accelerations [rad/s^2] x3 : Outport
  wires:
  Detect Change/1 -> Logical Operator5/1
  Difference/1 -> Gain/1
  Gain/1 -> Product/1
  Angular Velocities [rad/s] x3/1 -> Difference/1
  Logical Operator5/1 -> Product/2
  Enabled/1 -> Detect Change/1
  Product/1 -> Angular Accelerations [rad/s^2] x3/1

== system raibert_controller_walking/Behavior/Tranform Sensor Measurements to CoM Acceleration Measurement/Estimate Angular Accelerations3 ==
  Angular Velocities [rad/s] x2 : Inport
  Enabled : Inport  Port=2
  Detect Change : simulink/Logic and Bit Operations/Detect Change  vinit=0  OutDataTypeStr=boolean
  Difference : simulink/Discrete/Difference  ICPrevInput=0.0  OutMin=[]  OutMax=[]  OutDataType=fixdt(1, 16)  OutScaling=2^-10  DoSatur=off
  Gain : Gain  Gain=1/sample_time
  IMU Two Pole Filter : DiscreteTransferFcn  Commented=on  Numerator=[ctrl.A_lpf_lateral_accel 0 0]  Denominator=[1 ctrl.B1_lpf_lateral_accel ctrl.B2_lpf_lateral_accel]  SampleTime=sample_time
  Logical Operator5 : Logic  Operator=NOT  AllPortsSameDT=off  OutDataTypeStr=boolean
  Product : Product
  Angular Accelerations [rad/s^2] x2 : Outport
  wires:
  Enabled/1 -> Detect Change/1
  Logical Operator5/1 -> Product/2
  Angular Velocities [rad/s] x2/1 -> Difference/1
  Gain/1 -> Product/1
  Difference/1 -> Gain/1
  Detect Change/1 -> Logical Operator5/1
  Product/1 -> Angular Accelerations [rad/s^2] x2/1

== system raibert_controller_walking/Behavior/Filtering/Kalman Filtering/Subsystem ==
  right : Inport
  right? : Inport  Port=2
  left : Inport  Port=3
  Switch : Switch  Criteria=u2 ~= 0
  out : Outport
  wires:
  right/1 -> Switch/1
  right?/1 -> Switch/2
  left/1 -> Switch/3
  Switch/1 -> out/1

== system raibert_controller_walking/Behavior/Filtering/Kalman Filtering/Subsystem1 ==
  right : Inport
  right? : Inport  Port=2
  left : Inport  Port=3
  Switch : Switch  Criteria=u2 ~= 0
  out : Outport
  wires:
  right/1 -> Switch/1
  right?/1 -> Switch/2
  left/1 -> Switch/3
  Switch/1 -> out/1

== system raibert_controller_walking/Behavior/Filtering/Kalman Filtering/Subsystem2 ==
  right : Inport
  right? : Inport  Port=2
  left : Inport  Port=3
  Switch : Switch  Criteria=u2 ~= 0
  out : Outport
  wires:
  right/1 -> Switch/1
  right?/1 -> Switch/2
  left/1 -> Switch/3
  Switch/1 -> out/1

== matlab function raibert_controller_walking/Behavior/Swing Leg Control Secondary/Avoid Hitting Mechanical Limits ==
  data: back_cmd output double; front_cmd output double; dback_cmd output double; dfront_cmd output double; ddback_cmd output double; ddfront_cmd output double; back_desired input; dback_desired input; ddback_desired input; front_desired input; dfront_desired input; ddfront_desired input; ctrl parameter
%% Avoid fourbar limits by saturating the commands and ensuring we don't command velocities or 
% accelerations that would push us into the limits when nearby
function [back_cmd, front_cmd, dback_cmd, dfront_cmd, ddback_cmd, ddfront_cmd] ...
    = AvoidFourbarLimits(back_desired,dback_desired, ddback_desired, ...
          front_desired, dfront_desired, ddfront_desired, ...
          ctrl)
    [back_cmd, front_cmd, dback_cmd, dfront_cmd, ddback_cmd, ddfront_cmd] = ...
      AvoidFourbarLimits(back_desired, dback_desired, ddback_desired, ...
                         front_desired, dfront_desired, ddfront_desired, ...
                         ctrl.min_front_bar_angle, ctrl.max_front_bar_angle, ...
                         ctrl.min_back_bar_angle, ctrl.max_back_bar_angle);
end

== matlab function raibert_controller_walking/Behavior/2D Lateral Stance Control2 ==
  data: F_leg input; lateral_torque output; ctrl parameter
function lateral_torque = lateral_stance_control_on_boom(F_leg,ctrl)
    lateral_torque = F_leg*ctrl.lateral_offset*(ctrl.m_total-(ctrl.m_leg_motor+ctrl.m_leg))/ctrl.m_total;
end

== stateflow chart raibert_controller_walking/Behavior/Contact/Left Leg State ==
  state Stance
  state Twilight
  state Swing
  (junction 196) -> Stance
  (junction 198) -> (junction 196)
  Stance -> Twilight : [terminate_contact && force < touchdown_threshold]
  Twilight -> Swing : after(ctrl.twilight_time, sec)
  (default) -> Swing
  Swing -> (junction 198) : [force > touchdown_threshold]
  data: force input; touchdown_threshold input; ctrl parameter; Stance output boolean; Twilight output boolean; Swing output boolean; terminate_contact input

== matlab function raibert_controller_walking/Behavior/2D Lateral Stance Control3 ==
  data: F_leg input; lateral_torque output; ctrl parameter
function lateral_torque = lateral_stance_control_on_boom(F_leg,ctrl)
    lateral_torque = F_leg*ctrl.lateral_offset*(ctrl.m_total-(ctrl.m_leg_motor+ctrl.m_leg))/ctrl.m_total;
end

== matlab function raibert_controller_walking/Behavior/SEA Measurements/Leg Dynamics Right ==
  data: tau_back input; tau_front input; axial_force output; leg_width input; leg_length input; ortho_force output
function [axial_force, ortho_force] = fcn(tau_back, tau_front, leg_width, leg_length)

  % prevent divide by zero
  leg_width(1) = max(leg_width(1),eps);
  leg_length(1) = max(leg_length(1),eps);

  % forces and torques
  hip_torque = tau_front + tau_back;
  spread_torque = tau_front - tau_back;
  axial_force = zeros(2,1);
  axial_force(1) = spread_torque(1) / leg_width(1);
  ortho_force = zeros(2,1);
  ortho_force(1) = hip_torque(1) / leg_length(1);
  
  % time derivatives
  axial_force(2) = (leg_width(1)*spread_torque(2) - spread_torque(1)*leg_width(2)) / (leg_width(1)*leg_width(1));
  ortho_force(2) = (leg_length(1)*hip_torque(2) - hip_torque(1)*leg_length(2)) / (leg_length(1)*leg_length(1));
  
end

== stateflow chart raibert_controller_walking/Behavior/Contact/Right Leg State ==
  state Stance
  state Twilight
  state Swing
  (junction 196) -> Stance
  (junction 198) -> (junction 196)
  Stance -> Twilight : [terminate_contact && force < touchdown_threshold]
  Twilight -> Swing : after(ctrl.twilight_time, sec)
  (default) -> Swing
  Swing -> (junction 198) : [force > touchdown_threshold]
  data: force input; touchdown_threshold input; terminate_contact input; ctrl parameter; Stance output boolean; Twilight output boolean; Swing output boolean

== matlab function raibert_controller_walking/Behavior/Swing Leg Control Secondary/Convert CoM (X,Y,Z) to  (Leg Angles, Leg Length) ==
  data: desired_leg_length output; X_star input; Y_star input; Z_star input; right_left input; pelvis2com_pos input; desired_alpha output; desired_beta output; pelvis2com_vel input; roll input; pitch input; sagittal_angle input; lateral_angle input; leg_length input; ctrl parameter
%% Convert Foot2CoM vector from (X, Y, Z) to (leg length, leg angle) space
function [ desired_leg_length, desired_alpha, desired_beta ]  =  ...
          ConvertToJointAnglesAndLegLength(X_star, Y_star, Z_star, right_left,...
                           pelvis2com_pos, pelvis2com_vel, ...
                           roll, pitch, sagittal_angle, lateral_angle, leg_length,...
                           ctrl) 

    q = [roll(1), pitch(1), sagittal_angle(1), lateral_angle(1), leg_length(1)];
    dq = [roll(2), pitch(2), sagittal_angle(2), lateral_angle(2), leg_length(2)];
    [desired_alpha, desired_beta, desired_leg_length] = ...
      ConvertComPositionToLegAnglesAndLegLength(X_star, Y_star, Z_star, right_left, ...
                                                pelvis2com_pos, pelvis2com_vel, ...
                                                q, dq, ctrl.lateral_offset);
    desired_beta = saturate(desired_beta, ctrl.min_lateral_beta, ctrl.max_lateral_beta);
end

function [desired_saturated] = saturate(desired, min_lateral_beta, max_lateral_beta)
    desired_saturated = desired;
    if desired(1) < min_lateral_beta
        desired_saturated = [min_lateral_beta; 0; 0];
    elseif desired(1) > max_lateral_beta
        desired_saturated = [max_lateral_beta; 0; 0];    
    end
end
